simulink model "kyrs"  (R2021b)
settings: Solver=FixedStepAuto  StartTime=0.0  StopTime=100  FixedStep=0.01  MaxStep=1e-3  RelTol=1e-3
settings Model: Creator=pavel  LastModifiedBy=pavel

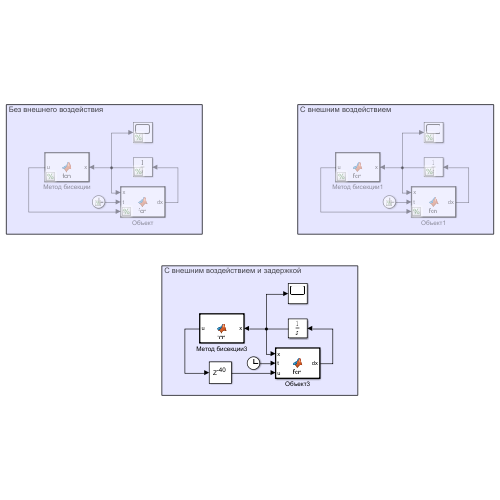
[thumbnail: Simulink's stored preview of the top-level diagram]
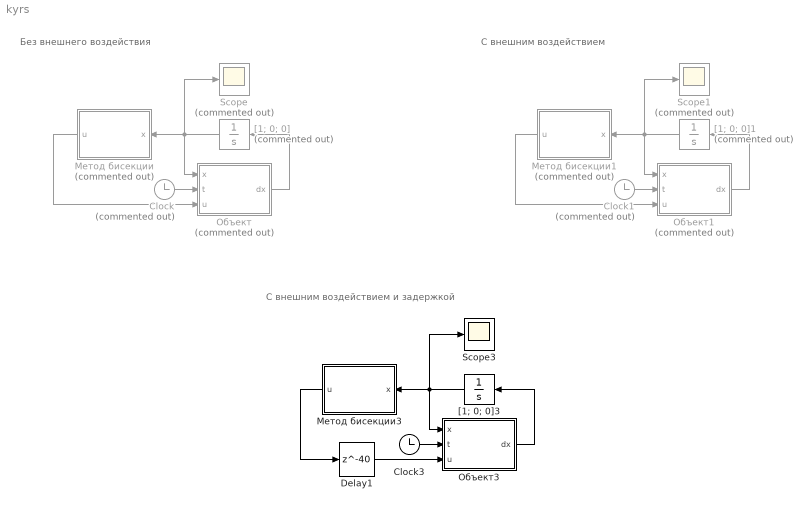
== system kyrs ==
  note: С внешним воздействием
  note: Без внешнего воздействия
  note: С внешним воздействием и задержкой
  Clock : Clock  Commented=on
  Clock1 : Clock  Commented=on
  Clock3 : Clock
  Delay1 : Delay  DelayLength=40
  Scope : Scope  Commented=on
  Scope1 : Scope  Commented=on
  Scope3 : Scope
  "[1; 0; 0]" : Integrator  Commented=on  InitialCondition=[1; 0; 0]
  "[1; 0; 0]1" : Integrator  Commented=on  InitialCondition=[1; 0; 0]
  "[1; 0; 0]3" : Integrator  InitialCondition=[1; 0; 0]
  Метод бисекции : MATLAB Function  Commented=on  TreatAsAtomicUnit=on
  Метод бисекции1 : MATLAB Function  Commented=on  TreatAsAtomicUnit=on
  Метод бисекции3 : MATLAB Function  TreatAsAtomicUnit=on
  Объект : MATLAB Function  Commented=on  TreatAsAtomicUnit=on
  Объект1 : MATLAB Function  Commented=on  TreatAsAtomicUnit=on
  Объект3 : MATLAB Function  TreatAsAtomicUnit=on
  wires:
  Clock/1 -> Объект/2(t)
  Объект/1(dx) -> "[1; 0; 0]"/1
  "[1; 0; 0]"/1 -> Метод бисекции/1(x), Scope/1, Объект/1(x)
  Метод бисекции/1(u) -> Объект/3(u)
  Метод бисекции1/1(u) -> Объект1/3(u)
  "[1; 0; 0]1"/1 -> Scope1/1, Объект1/1(x), Метод бисекции1/1(x)
  Объект1/1(dx) -> "[1; 0; 0]1"/1
  Clock1/1 -> Объект1/2(t)
  Clock3/1 -> Объект3/2(t)
  Объект3/1(dx) -> "[1; 0; 0]3"/1
  "[1; 0; 0]3"/1 -> Метод бисекции3/1(x), Объект3/1(x), Scope3/1
  Метод бисекции3/1(u) -> Delay1/1
  Delay1/1 -> Объект3/3(u)

== matlab function kyrs/Метод бисекции ==
  data: x input; u output
function u = fcn(x)
k = [-6.67328197345670	-10.7713543596927	-3.05149663828592];
P = [1.25520917793637e-08	1.32739293126156e-08	2.44164511041642e-09
1.32739293126156e-08	2.11072417695046e-08	4.21465980112481e-09
2.44164511041642e-09	4.21465980112481e-09	2.71143732800415e-09];
mu=1/2;
alpha=1;
gamma=4.5;
Vmin = 0.01;
a = Vmin;
V0 = 1;
b = 1;
Da = [a^((-1)*(1+2*mu)) 0 0; 0 a^((-1)*(1+1*mu)) 0; 0 0 a^(-1)];
Db = [b^((-1)*(1+2*mu)) 0 0; 0 b^((-1)*(1+1*mu)) 0; 0 0 b^(-1)];
for i=1:1:10
if (x'*Db*P*Db*x>1)
    a=b;b=2*b;
elseif (x'*Da*P*Da*x<1)
    b=a;a=max(a/2,Vmin);
else
    c=(a+b)/2;
    Dc = [c^((-1)*(1+2*mu)) 0 0; 0 c^((-1)*(1+1*mu)) 0; 0 0 c^(-1)];
    if(x'*Dc*P*Dc*x<1)
        b=c;
    else
        a=max(c,Vmin);
    end
end
end
V = b;
DV = [V^((-1)*(1+2*mu)) 0 0; 0 V^((-1)*(1+1*mu)) 0; 0 0 V^(-1)];
u = V^(1-mu)*k*DV*x;

== matlab function kyrs/Объект ==
  data: x input; dx output; t input; u input
function dx  = fcn(x, t, u)
dx = x;
A = [0 1 0; 0 0 1; 0 0 0];
b = [0; 0; 1];
dx = A*x + b*u;

== matlab function kyrs/Метод бисекции1 ==
  data: x input; u output
function u = fcn(x)
k = [-0.199143859581487	-0.934296071578915	-1.47866293081497];
P = [0.103366111497637	0.343876533665082	0.348565132196896
0.343876533665082	1.36768925390524	1.50512104097002
0.348565132196896	1.50512104097002	2.24287767009687];
mu=1;
alpha=0.6;
beta=0.3;
gamma=7.5;
Vmin = 0.1;
u0=1;
a = Vmin;
V0 = 1;
b = 1;
Da = [a^((-1)*(1+2*mu)) 0 0; 0 a^((-1)*(1+1*mu)) 0; 0 0 a^(-1)];
Db = [b^((-1)*(1+2*mu)) 0 0; 0 b^((-1)*(1+1*mu)) 0; 0 0 b^(-1)];
for i=1:1:10
if (x'*Db*P*Db*x>1)
    a=b;b=2*b;
elseif (x'*Da*P*Da*x<1)
    b=a;a=max(a/2,Vmin);
else
    c=(a+b)/2;
    Dc = [c^((-1)*(1+2*mu)) 0 0; 0 c^((-1)*(1+1*mu)) 0; 0 0 c^(-1)];
    if(x'*Dc*P*Dc*x<1)
        b=c;
    else
        a=max(c,Vmin);
    end
end
end
V = b;
DV = [V^((-1)*(1+2*mu)) 0 0; 0 V^((-1)*(1+1*mu)) 0; 0 0 V^(-1)];
u = V^(1-mu)*k*DV*x;

== matlab function kyrs/Объект1 ==
  data: x input; dx output; t input; u input
function dx  = fcn(x, t, u)
dx = x;
A = [0 1 0; 0 0 1; 0 0 0];
b = [0; 0; 1];
betta = [0; 0; 0.3*sin(t)];
dx = A*x + b*u + betta'*x;

== matlab function kyrs/Метод бисекции3 ==
  data: x input; u output
function u = fcn(x)
k = [-0.199143859581487	-0.934296071578915	-1.47866293081497];
P = [0.103366111497637	0.343876533665082	0.348565132196896
0.343876533665082	1.36768925390524	1.50512104097002
0.348565132196896	1.50512104097002	2.24287767009687];
mu=1;
alpha=0.6;
beta=0.3;
gamma=7.5;
Vmin = 0.1;
u0=1;
a = Vmin;
V0 = 1;
b = 1;
Da = [a^((-1)*(1+2*mu)) 0 0; 0 a^((-1)*(1+1*mu)) 0; 0 0 a^(-1)];
Db = [b^((-1)*(1+2*mu)) 0 0; 0 b^((-1)*(1+1*mu)) 0; 0 0 b^(-1)];
for i=1:1:10
if (x'*Db*P*Db*x>1)
    a=b;b=2*b;
elseif (x'*Da*P*Da*x<1)
    b=a;a=max(a/2,Vmin);
else
    c=(a+b)/2;
    Dc = [c^((-1)*(1+2*mu)) 0 0; 0 c^((-1)*(1+1*mu)) 0; 0 0 c^(-1)];
    if(x'*Dc*P*Dc*x<1)
        b=c;
    else
        a=max(c,Vmin);
    end
end
end
V = b;
DV = [V^((-1)*(1+2*mu)) 0 0; 0 V^((-1)*(1+1*mu)) 0; 0 0 V^(-1)];
u = V^(1-mu)*k*DV*x;

== matlab function kyrs/Объект3 ==
  data: x input; dx output; t input; u input
function dx  = fcn(x, t, u)
dx = x;
A = [0 1 0; 0 0 1; 0 0 0];
b = [0; 0; 1];
betta = [0; 0; 0.3*sin(t)];
dx = A*x + b*u + betta'*x;
